simulink model "fxpdemo_state_space"  (Simulink 5.0)
settings: Solver=ode5  SolverMode=SingleTasking  StartTime=0.0  StopTime=2  FixedStep=SampleTime/5  RelTol=1e-3  AbsTol=1e-6
PreLoadFcn:
  | preload_state_space
InitFcn:
  | ;
StartFcn:
  | ;
StopFcn:
  | ;
values from neighbouring files (symbols this model uses):
  Ab_z = [0.967403570605  0.170823854812  -0.0242324942444; -0.170823854812  0.926222958366  0.0877139172259; -0.0242324942444  -0.0877139172259  0.810269574925]    [preload_state_space.mat]
  Ac_s = [-28  -17.5  -15.625; 32  0  0; 0  16  0]    [preload_state_space.mat]
  Ac_z = [2.7038961039  -1.23333333333  0.755844155844; 2  0  0; 0  0.5  0]    [preload_state_space.mat]
  Bb_z = [0.464411605731 0.584624602794 0.381918236531]    [preload_state_space.mat]
  Bc_s = [8 0 0]    [preload_state_space.mat]
  Bc_z = [0.125 0 0]    [preload_state_space.mat]
  Cb_z = [0.464411605731 -0.584624602794 0.381918236531]    [preload_state_space.mat]
  Cc_s = [0 0 7.8125]    [preload_state_space.mat]
  Cc_z = [0.158030021926 0.00738816738817 0.0486467644909]    [preload_state_space.mat]
  Db_z = 0.0034632034632    [preload_state_space.mat]
  Dc_s = 0    [preload_state_space.mat]
  Dc_z = 0.0034632034632    [preload_state_space.mat]
  SampleTime = 0.05    [preload_diff.m]    (also in preload_state_space.mat = 0.01)
  xb0_z = [0 0 0]    [preload_state_space.mat]
  xc0_s = [0 0 0]    [preload_state_space.mat]
  xc0_z = [0 0 0]    [preload_state_space.mat]
libraries: fixpt_lib_4 x6, fixpt_lib_3p1 x1
PreSaveFcn:
  | ;
settings Model: CovMetricSettings=d  MinMaxOverflowLogging=MinMaxAndOverflow  Creator=andyb  LastModifiedBy=andyb  ExtModeTrigMode=oneshot  ExtModeArmWhenConnect=off  ExtModeAutoUpdateStatusClock=off  RTWExpressionDepthLimit=1  LimitDataPoints=off  IntegerOverflowMsg=none  ParameterDowncastMsg=warning  ParameterOverflowMsg=warning  ParameterPrecisionLossMsg=none  RTWInlineParameters=on  RTWOptions="-aEnforceIntegerDowncast=1 -aExtMode=0 -aExtModeTesting=0 -aFoldNonRolledExpr=1 -aForceParamTrailComments=0 -aGenerateComments=1 -aGenerateReport=1 -aIgnoreCustomStorageClasses=1 -aIncDataTypeInIds=0 -aIncHierarchyInIds=0 -aInlineInvariantSignals=0 -aInlinedPrmAccess=\"Literals\" -aLocalBlockOutputs=1 -aLogVarNameModifier=\"rt_\" -aMaxRTWIdLen=31 -aPrefixModelToSubsysFcnNames=1 -aRTWVerbose=1 -aRollThreshold=5 -aShowEliminatedStatements=0"

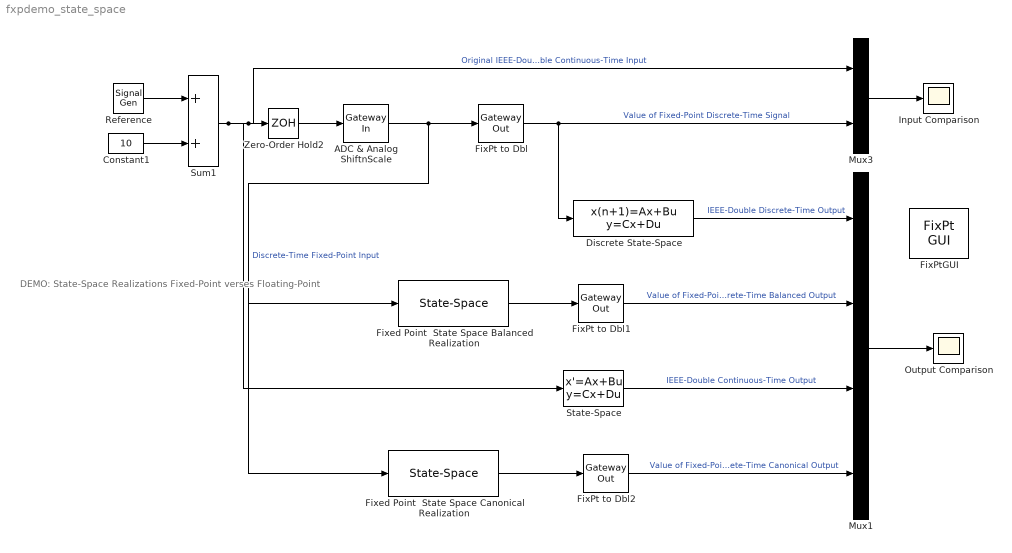
== system fxpdemo_state_space ==
  note: DEMO:
      |
      | State-Space
      | Realizations
      |
      | Fixed-Point
      | verses
      | Floating-Point
  ADC & Analog ShiftnScale : fixpt_lib_4/Data Type/Gateway In  InRealWorld=Real World Value  OutputDataTypeScalingMode=Specify via dialog  OutDataType=BaseType  OutScaling=2^-6  RndMeth=Nearest  DoSatur=on
      settings: LockScale=on
  Constant1 : Constant  Value=10
  Discrete State-Space : DiscreteStateSpace  A=Ac_z  B=Bc_z  C=Cc_z  D=Dc_z  X0=xc0_z  SampleTime=SampleTime
  FixPt to Dbl : fixpt_lib_4/Data Type/Gateway Out  OutRealWorld=Real World Value  OutBuiltInType=double  DoSatur=off
  FixPt to Dbl1 : fixpt_lib_4/Data Type/Gateway Out  OutRealWorld=Real World Value  OutBuiltInType=double  DoSatur=off
  FixPt to Dbl2 : fixpt_lib_4/Data Type/Gateway Out  OutRealWorld=Real World Value  OutBuiltInType=double  DoSatur=off
  FixPtGUI : fixpt_lib_3p1/FixPt GUI
  Fixed Point  State Space Balanced Realization : fixpt_lib_4/Filters/State-Space  A=Ab_z  B=Bb_z  C=Cb_z  D=Db_z  X0=xb0_z  InternalDataType=LongType  StateEqScaling=2^(-14)  OutputEqScaling=2^(-15)  DoSatur=off
  Fixed Point  State Space Canonical Realization : fixpt_lib_4/Filters/State-Space  A=Ac_z  B=Bc_z  C=Cc_z  D=Dc_z  X0=xc0_z  InternalDataType=LongType  StateEqScaling=2^(-12)  OutputEqScaling=2^(-15)  DoSatur=off
  Input Comparison : Scope
      settings: TickLabels=on  YMin=-10  YMax=30  SaveName=InputComparison
  Mux1 : Mux
  Mux3 : Mux  Inputs=2
  Output Comparison : Scope
      settings: TickLabels=on  TimeRange=2  YMin=-60  YMax=140  SaveName=OutputComparison
  Reference : SignalGenerator  WaveForm=square  Amplitude=-10  Frequency=0.5
  State-Space : StateSpace  A=Ac_s  B=Bc_s  C=Cc_s  D=Dc_s  X0=xc0_s
  Sum1 : Sum  Inputs=2  SaturateOnIntegerOverflow=on  InputSameDT=on
  Zero-Order Hold2 : ZeroOrderHold  SampleTime=SampleTime
  wires:
  Reference/1 -> Sum1/1
  Constant1/1 -> Sum1/2
  Sum1/1 -> Mux3/1, State-Space/1, Zero-Order Hold2/1  "Original IEEE-Double Continuous-Time Input"
  Zero-Order Hold2/1 -> ADC & Analog ShiftnScale/1
  ADC & Analog ShiftnScale/1 -> FixPt to Dbl/1, Fixed Point  State Space Balanced Realization/1, Fixed Point  State Space Canonical Realization/1  "Discrete-Time Fixed-Point Input"
  FixPt to Dbl/1 -> Mux3/2, Discrete State-Space/1  "Value of Fixed-Point Discrete-Time Signal"
  Fixed Point  State Space Canonical Realization/1 -> FixPt to Dbl2/1
  FixPt to Dbl1/1 -> Mux1/2  "Value of Fixed-Point Discrete-Time Balanced Output"
  Fixed Point  State Space Balanced Realization/1 -> FixPt to Dbl1/1
  State-Space/1 -> Mux1/3  "IEEE-Double Continuous-Time Output"
  Discrete State-Space/1 -> Mux1/1  "IEEE-Double Discrete-Time Output"
  FixPt to Dbl2/1 -> Mux1/4  "Value of Fixed-Point Discrete-Time Canonical Output"
  Mux1/1 -> Output Comparison/1
  Mux3/1 -> Input Comparison/1
